simulink library "GFL_Lib"  (R2021a)
settings: Solver=VariableStepAuto  StartTime=0.0  StopTime=10.0  RelTol=1e-3
values from neighbouring files (symbols this model uses):
  Ki_i = 0    [Init_GFL.m]
  Kp_i = Lc_eq/wb*wn_i    [Init_GFL.m]
  Kp_Rvi_pu = X_VI/(DX_DR*(I_Max_TVI_pu-1))    [Init_GFM.m]
  Lc_eq = Lc_pu + dLc_pu    [Init_VI.m]    (also in Init_VI_mmc.m)
  Lc_pu = Lt_pu    [Init_VI.m]    (also in Init_VI_mmc.m = Lt_pu+Larm_pu/2)
  Lf_pu = Lc_eq    [Init_GFL.m]
  Va0 = Vm0*sqrt(2)*Vb1*sin(Theta_Vm0*pi/180)    [Init_LF_L.m]    (also in Init_LF_MMC.m)
  Vb0 = Vm0*sqrt(2)*Vb1*sin(Theta_Vm0*pi/180-2*pi/3)    [Init_LF_L.m]    (also in Init_LF_MMC.m)
  Vc0 = Vm0*sqrt(2)*Vb1*sin(Theta_Vm0*pi/180+2*pi/3)    [Init_LF_L.m]    (also in Init_LF_MMC.m)
  Vm0 = abs(V1)    [Init_LF_L.m]    (also in Init_LF_MMC.m)
  Vm0_d = Vvsc0*cos(angle(Vvirt))    [Init_LF_L.m]    (also in Init_LF_MMC.m)
  Vm0_q = Vvsc0*sin(angle(Vvirt))    [Init_LF_L.m]    (also in Init_LF_MMC.m)
  Vvsc0 = abs(Vvirt)    [Init_LF_L.m]    (also in Init_LF_MMC.m)
undefined symbols (not defined in the file or in its folder): Carm, Diff_CC_ki, Diff_CC_kp, fb, Ib2, Idcb, Ki_Wdiff_pu, Ki_Wtot_pu, Kp_Wdiff_pu, Kp_Wtot_pu, Lb, Sb, Solver_Time_Step, Time_Step, Vb1, Vb2, Vdcb, VSC01_id0, wb, Zb
libraries: Control_Lib x57, spsVoltageMeasurementLib x17, spsSeriesRLCBranchLib x14, spsThreePhaseSourceLib x12, spsThreePhaseBreakerLib x10, spsThreePhaseVIMeasurementLib x9, spsThreePhaseTransformerTwoWindingsLib x7, spsCurrentMeasurementLib x7, powerlib x7, spsControlledCurrentSourceLib x6, spsControlledVoltageSourceLib x6, slpidlib x6
(part 6 of 6)

== system GFL_Lib/Mean Model 2-Level L-filter_old/Control loops/Inner Current Control/Current PI control/PI_fw_init ==
  Ref : Inport
  Meas : Inport  Port=2
  fw : Inport  Port=3
  y0 : Inport  Port=4
  held_integ : Inport  Port=5
  Constant : Constant  Value=0
  Constant1 : Constant  Value=0
  Data Type Conversion : DataTypeConversion
  Gain : Gain  Gain=Kp
  Gain1 : Gain  Gain=Ki
  Init_condition : Subsystem
  Integrator : Integrator  InitialConditionSource=external
  Memory : Memory  InitialCondition=1
  Subsystem : Subsystem  Commented=on
  Sum : Sum
  Sum1 : Sum  Inputs=+-
  Sum2 : Sum
  Switch : Switch  Criteria=u2 > Threshold  Threshold=0.5
  y : Outport  VectorParamsAs1DForOutWhenUnconnected=off
  wires:
  Init_condition/1(integ0) -> Integrator/2
  [comp] -> Init_condition/2(comp)
  Ref/1 -> Sum1/1
  Meas/1 -> Sum1/2
  Sum/1 -> Sum2/1, [comp]
  Sum1/1 -> Gain/1, Gain1/1
  Sum2/1 -> y/1
  y0/1 -> Init_condition/1(y0)
  Constant/1 -> Memory/1
  Memory/1 -> Init_condition/Enable
  fw/1 -> Sum/1
  Gain/1 -> Sum/2
  Integrator/1 -> Sum2/2
  Switch/1 -> Integrator/1
  Constant1/1 -> Switch/1
  Gain1/1 -> Switch/3
  held_integ/1 -> Data Type Conversion/1
  Data Type Conversion/1 -> Switch/2

== system GFL_Lib/Mean Model 2-Level L-filter_old/Control loops/Inner Current Control/Current PI control/PI_fw_init1 ==
  Ref : Inport
  Meas : Inport  Port=2
  fw : Inport  Port=3
  y0 : Inport  Port=4
  held_integ : Inport  Port=5
  Constant : Constant  Value=0
  Constant1 : Constant  Value=0
  Data Type Conversion : DataTypeConversion
  Gain : Gain  Gain=Kp
  Gain1 : Gain  Gain=Ki
  Init_condition : Subsystem
  Integrator : Integrator  InitialConditionSource=external
  Memory : Memory  InitialCondition=1
  Subsystem : Subsystem  Commented=on
  Sum : Sum
  Sum1 : Sum  Inputs=+-
  Sum2 : Sum
  Switch : Switch  Criteria=u2 > Threshold  Threshold=0.5
  y : Outport  VectorParamsAs1DForOutWhenUnconnected=off
  wires:
  Init_condition/1(integ0) -> Integrator/2
  [comp] -> Init_condition/2(comp)
  Ref/1 -> Sum1/1
  Meas/1 -> Sum1/2
  Sum/1 -> Sum2/1, [comp]
  Sum1/1 -> Gain/1, Gain1/1
  Sum2/1 -> y/1
  y0/1 -> Init_condition/1(y0)
  Constant/1 -> Memory/1
  Memory/1 -> Init_condition/Enable
  fw/1 -> Sum/1
  Gain/1 -> Sum/2
  Integrator/1 -> Sum2/2
  Switch/1 -> Integrator/1
  Constant1/1 -> Switch/1
  Gain1/1 -> Switch/3
  held_integ/1 -> Data Type Conversion/1
  Data Type Conversion/1 -> Switch/2

== system GFL_Lib/Mean Model 2-Level L-filter with DC Link/Control loops/Inner Current Control/Current PI control/PI_fw_init/Init_condition ==
  y0 : Inport
  comp : Inport  Port=2
  Enable : EnablePort
  Sum : Sum  Inputs=-+
  integ0 : Outport  VectorParamsAs1DForOutWhenUnconnected=off
  wires:
  Sum/1 -> integ0/1
  y0/1 -> Sum/2
  comp/1 -> Sum/1

== system GFL_Lib/Mean Model 2-Level L-filter with DC Link/Control loops/Inner Current Control/Current PI control/PI_fw_init/Subsystem ==
  e : Inport
  x0 : Inport  Port=2
  Enable : EnablePort
  Integrator : Integrator  InitialConditionSource=external
  y : Outport  VectorParamsAs1DForOutWhenUnconnected=off
  wires:
  x0/1 -> Integrator/2
  Integrator/1 -> y/1
  e/1 -> Integrator/1

== system GFL_Lib/Mean Model 2-Level L-filter with DC Link/Control loops/Inner Current Control/Current PI control/PI_fw_init1/Init_condition ==
  y0 : Inport
  comp : Inport  Port=2
  Enable : EnablePort
  Sum : Sum  Inputs=-+
  integ0 : Outport  VectorParamsAs1DForOutWhenUnconnected=off
  wires:
  Sum/1 -> integ0/1
  y0/1 -> Sum/2
  comp/1 -> Sum/1

== system GFL_Lib/Mean Model 2-Level L-filter with DC Link/Control loops/Inner Current Control/Current PI control/PI_fw_init1/Subsystem ==
  e : Inport
  x0 : Inport  Port=2
  Enable : EnablePort
  Integrator : Integrator  InitialConditionSource=external
  y : Outport  VectorParamsAs1DForOutWhenUnconnected=off
  wires:
  x0/1 -> Integrator/2
  Integrator/1 -> y/1
  e/1 -> Integrator/1

== system GFL_Lib/Mean Model 2-Level L-filter_old/Control loops/Inner Current Control/Current PI control/PI_fw_init/Init_condition ==
  y0 : Inport
  comp : Inport  Port=2
  Enable : EnablePort
  Sum : Sum  Inputs=-+
  integ0 : Outport  VectorParamsAs1DForOutWhenUnconnected=off
  wires:
  Sum/1 -> integ0/1
  y0/1 -> Sum/2
  comp/1 -> Sum/1

== system GFL_Lib/Mean Model 2-Level L-filter_old/Control loops/Inner Current Control/Current PI control/PI_fw_init/Subsystem ==
  e : Inport
  x0 : Inport  Port=2
  Enable : EnablePort
  Integrator : Integrator  InitialConditionSource=external
  y : Outport  VectorParamsAs1DForOutWhenUnconnected=off
  wires:
  x0/1 -> Integrator/2
  Integrator/1 -> y/1
  e/1 -> Integrator/1

== system GFL_Lib/Mean Model 2-Level L-filter_old/Control loops/Inner Current Control/Current PI control/PI_fw_init1/Init_condition ==
  y0 : Inport
  comp : Inport  Port=2
  Enable : EnablePort
  Sum : Sum  Inputs=-+
  integ0 : Outport  VectorParamsAs1DForOutWhenUnconnected=off
  wires:
  Sum/1 -> integ0/1
  y0/1 -> Sum/2
  comp/1 -> Sum/1

== system GFL_Lib/Mean Model 2-Level L-filter_old/Control loops/Inner Current Control/Current PI control/PI_fw_init1/Subsystem ==
  e : Inport
  x0 : Inport  Port=2
  Enable : EnablePort
  Integrator : Integrator  InitialConditionSource=external
  y : Outport  VectorParamsAs1DForOutWhenUnconnected=off
  wires:
  x0/1 -> Integrator/2
  Integrator/1 -> y/1
  e/1 -> Integrator/1
